simulink model "model"  (R2022a)
settings: Solver=VariableStepAuto  StartTime=0.0  StopTime=10.0  RelTol=1e-3
settings Model: Creator=zachk  LastModifiedBy=zachk

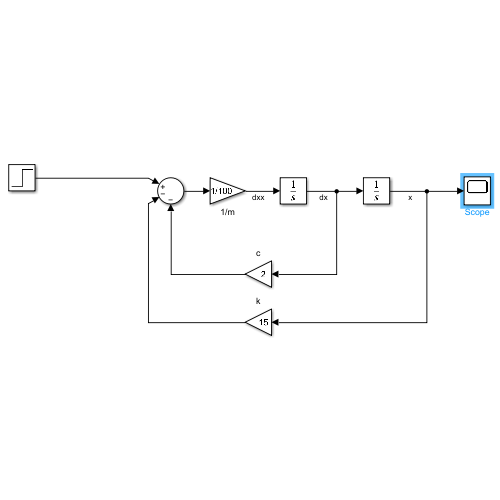
[thumbnail: Simulink's stored preview of the top-level diagram]
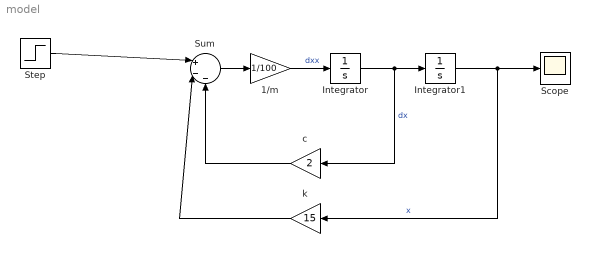
== system model ==
  1/m : Gain  Gain=1/100
  Integrator : Integrator
  Integrator1 : Integrator
  Scope : Scope
  Step : Step  SampleTime=0
  Sum : Sum  Inputs=|+--
  c : Gain  Gain=2
  k : Gain  Gain=15
  wires:
  c/1 -> Sum/3
  k/1 -> Sum/2
  Sum/1 -> 1/m/1
  1/m/1 -> Integrator/1  "dxx"
  Integrator/1 -> c/1, Integrator1/1  "dx"
  Integrator1/1 -> k/1, Scope/1  "x"
  Step/1 -> Sum/1
